simulink model "tocdo1"  (R2018b)
settings: Solver=FixedStepAuto  StartTime=0.0  StopTime=2  FixedStep=0.0002  RelTol=1e-3
undefined symbols (not defined in the file): J, KE, OmegaN, Tf, Tsp, Zeta
settings Model: Creator=User  LastModifiedBy=User

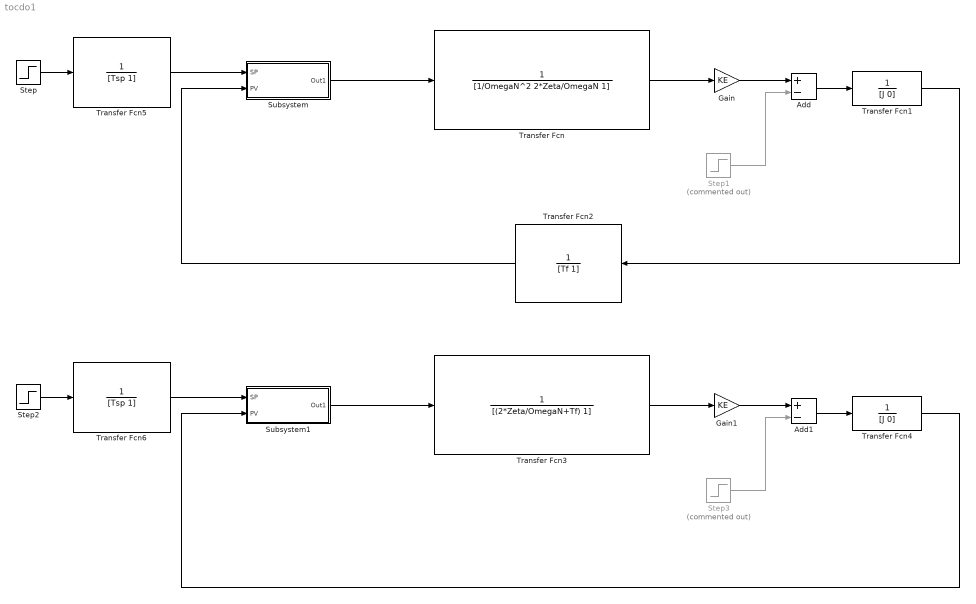
== system tocdo1 ==
  Add : Sum  Inputs=+-
  Add1 : Sum  Inputs=+-
  Gain : Gain  Gain=KE
  Gain1 : Gain  Gain=KE
  Step : Step  Time=0  After=1000  SampleTime=0
  Step1 : Step  Commented=on  Time=0.5  After=70  SampleTime=0
  Step2 : Step  Time=0  After=1000  SampleTime=0
  Step3 : Step  Commented=on  Time=0.5  After=70  SampleTime=0
  Subsystem : Subsystem
  Subsystem1 : Subsystem
  Transfer Fcn : TransferFcn  Denominator=[1/OmegaN^2 2*Zeta/OmegaN 1]
  Transfer Fcn1 : TransferFcn  Denominator=[J 0]
  Transfer Fcn2 : TransferFcn  Denominator=[Tf 1]
  Transfer Fcn3 : TransferFcn  Denominator=[(2*Zeta/OmegaN+Tf) 1]
  Transfer Fcn4 : TransferFcn  Denominator=[J 0]
  Transfer Fcn5 : TransferFcn  Denominator=[Tsp 1]
  Transfer Fcn6 : TransferFcn  Denominator=[Tsp 1]
  wires:
  Transfer Fcn/1 -> Gain/1
  Gain/1 -> Add/1
  Add/1 -> Transfer Fcn1/1
  Subsystem/1(Out1) -> Transfer Fcn/1
  Step/1 -> Transfer Fcn5/1
  Transfer Fcn1/1 -> Transfer Fcn2/1
  Step1/1 -> Add/2
  Transfer Fcn2/1 -> Subsystem/2(PV)
  Transfer Fcn4/1 -> Subsystem1/2(PV)
  Step3/1 -> Add1/2
  Step2/1 -> Transfer Fcn6/1
  Subsystem1/1(Out1) -> Transfer Fcn3/1
  Add1/1 -> Transfer Fcn4/1
  Gain1/1 -> Add1/1
  Transfer Fcn3/1 -> Gain1/1
  Transfer Fcn5/1 -> Subsystem/1(SP)
  Transfer Fcn6/1 -> Subsystem1/1(SP)

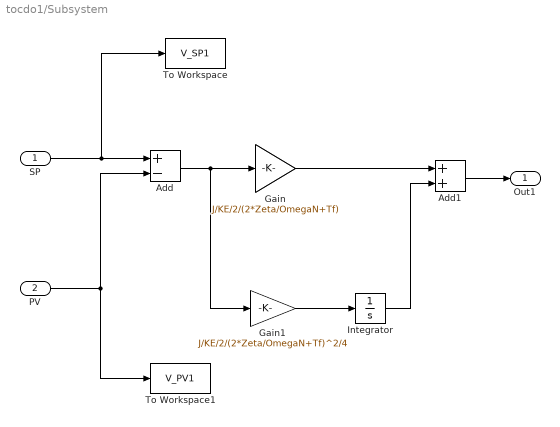
== system tocdo1/Subsystem ==
  SP : Inport
  PV : Inport  Port=2
  Add : Sum  Inputs=+-
  Add1 : Sum
  Gain : Gain  Gain=J/KE/2/(2*Zeta/OmegaN+Tf)
  Gain1 : Gain  Gain=J/KE/2/(2*Zeta/OmegaN+Tf)^2/4
  Integrator : Integrator
  To Workspace : ToWorkspace  VariableName=V_SP1  SaveFormat=Timeseries  SampleTime=-1
  To Workspace1 : ToWorkspace  VariableName=V_PV1  SaveFormat=Timeseries  SampleTime=-1
  Out1 : Outport
  wires:
  SP/1 -> To Workspace/1, Add/1
  PV/1 -> Add/2, To Workspace1/1
  Add/1 -> Gain1/1, Gain/1
  Gain1/1 -> Integrator/1
  Gain/1 -> Add1/1
  Integrator/1 -> Add1/2
  Add1/1 -> Out1/1

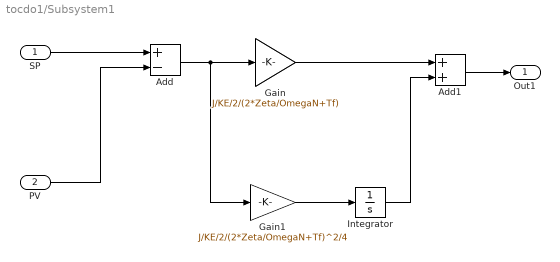
== system tocdo1/Subsystem1 ==
  SP : Inport
  PV : Inport  Port=2
  Add : Sum  Inputs=+-
  Add1 : Sum
  Gain : Gain  Gain=J/KE/2/(2*Zeta/OmegaN+Tf)
  Gain1 : Gain  Gain=J/KE/2/(2*Zeta/OmegaN+Tf)^2/4
  Integrator : Integrator
  Out1 : Outport
  wires:
  Add1/1 -> Out1/1
  Integrator/1 -> Add1/2
  Gain/1 -> Add1/1
  Gain1/1 -> Integrator/1
  Add/1 -> Gain/1, Gain1/1
  PV/1 -> Add/2
  SP/1 -> Add/1
